simulink library "DCAC_Converter"  (R2018b)
settings: Solver=VariableStepAuto  StartTime=0.0  StopTime=10.0  RelTol=1e-3
settings Model: Creator=Tony  LastModifiedBy=ga69qig
settings SFSimCC: SimUseLocalCustomCode=off
settings RTWCC: RTWUseLocalCustomCode=off

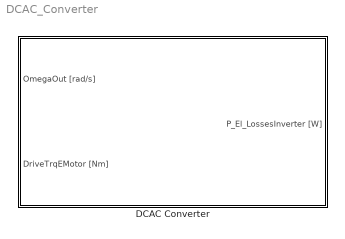
== system DCAC_Converter ==
  DCAC Converter : Subsystem  mask(SB){W_Vektor=[0 10.4719755119660 21.7817090648892 33.0914426178125 44.4011761707357 55.7109097236590 67.0206432765823 78.3303768295055 89.6401103824288 100.949843935352 112.259577488275 123.569311041199 134.879044594122 146.188778147045 157.498511699968 168.808245252892 180.117978805815 191.427712358738 202.737445911661 214.047179464585 225.356913017508 236.666646570431 247.976380123354 259.286113676278 270.595847229201 281.905580782124 293.215314335047 304.525047887971 315.834781440894 327.144514993817 338.454248546740 349.763982099664 361.073715652587 372.383449205510 383.693182758433 395.002916311357 406.312649864280 417.622383417203 428.932116970126 440.241850523050 451.551584075973 462.861317628896 474.171051181819 485.480784734743 496.790518287666 508.100251840589 519.409985393512 530.719718946436 542.029452499359 553.339186052282 564.648919605206 575.958653158129 587.268386711052 598.578120263975 609.887853816898 621.197587369822 632.507320922745 643.817054475668 655.126788028592 666.436521581515 677.746255134438], M_Vektor_motgen=[0 1 2 3 4 5 6 7 8 9 10 11 12 13 14 15 16 17 18 19 20 21 22 23 24 25 26 27 28 29 30 31 32 33 34 35 36 37 38 39 40 41 42 43 44 45 46 47 48 49 50 51 52 53 54 55 56 57 58 59 60 61 62 63 64 65 66 67 68 69 70 71 72 73 74 75 76 77 78 79 80 81 82 83 84 85 86 87 88 89 90 91 92 93 94 95 96 97 98 99 100 101 102 103 104 105 106 107 108 109 110 111 112 113 114 115 116 117 118 119 120 121 122 123 124 125 126 127 128 129 130], P_Loss=[0 0 0 0 0 0 0 0 0 0 0 0 0 0 0 0 0 0 0 0 0 0 0 0 0 0 0 0 0 0 0 0 0 0 0 0 0 0 0 0 0 0 0 0 0 0 0 0 0 0 0 0 0 0 0 0 0 0 0 0 0 0 0 0 0 0 0 0 0 0 0 0 0 0 0 0 0 0 0 0 0 0 0 0 0 0 0 0 0 0 0 0 0 0 0 0 0 0 0 0 0 0 0 0 0 0 0 0 0 0 0 0 0 0 0 0 0 0 0 0 0 0 0 0 0 0 0 0 0 0 0;0 82 70 84 90 100 106 112 101 115 122 130 144 146 153 162 154 169 188 198 202 216 231 236 247 260 271 279 293 309 316 326 335 353 373 392 407 427 437 460 475 478 493 505 523 529 551 565 570 582 598 616 631 647 665 682 700 716 730 726 743 763 780 805 824 840 861 884 903 919 947 960 981 995 1018 1041 1062 1086 1110 1130 1152 1170 1188 1211 1237 1259 1280 1302 1323 1344 1369 1392 1412 1440 1460 1493 1518 1540 1568 1594 1617 1646 1670 1709 1743 1769 1791 1825 1856 1881 1938 2212 3001 3444 3441 3510 3626 3825 3876 3879 3957 4140 4177 3954 4094 3971 3839 3839 3839 3839 3839;0 61 78 75 74 73 81 94 94 97 96 106 120 131 139 145 154 169 180 188 198 206 215 230 242 254 265 268 286 302 306 318 344 370 384 399 410 423 438 458 483 500 512 520 528 539 554 573 589 600 614 632 645 655 678 691 714 720 739 748 763 777 787 809 833 829 860 887 913 937 949 962 976 988 1007 1032 1049 1076 1095 1118 1143 1168 1192 1212 1231 1256 1293 1323 1337 1356 1387 1406 1427 1456 1469 1496 1515 1558 1577 1607 1643 1675 1694 1710 1739 1772 1805 1832 1870 1893 1924 1942 1976 1999 2049 2640 3767 4034 4108 4084 4241 4351 4407 4486 4544 4620 3839 3839 3839 3839 3839;0 70 71 95 83 94 92 96 105 107 112 125 141 143 150 153 165 176 190 203 218 233 240 245 253 260 274 285 304 329 341 352 358 365 379 403 424 444 460 472 483 499 525 535 543 561 575 589 597 611 632 643 656 664 677 700 719 731 742 759 777 794 814 839 858 870 892 917 938 953 968 987 1008 1022 1035 1055 1085 1111 1129 1151 1176 1192 1213 1240 1276 1296 1325 1348 1369 1387 1405 1432 1465 1493 1507 1525 1558 1586 1614 1642 1663 1683 1718 1753 1777 1801 1832 1860 1893 1925 1956 1984 2007 2030 2062 2093 2124 2160 2187 2222 2252 2304 2714 4353 4916 3997 3839 3839 3839 3839 3839;0 74 50 130 190 192 101 114 128 71 125 147 164 97 157 185 186 201 216 227 232 238 241 252 264 279 293 306 320 335 355 350 365 394 396 405 423 436 452 468 481 497 508 518 532 545 554 569 588 604 613 625 645 667 677 690 709 726 745 765 780 791 803 829 843 855 881 897 912 926 942 967 994 1017 1036 1056 1073 1104 1121 1152 1181 1210 1240 1264 1282 1303 1323 1349 1371 1396 1415 1439 1469 1495 1515 1540 1563 1591 1625 1648 1677 1706 1736 1764 1793 1824 1842 1877 1912 1945 1975 2002 2024 2048 2081 2116 2143 2180 2207 2259 2278 2340 2348 2402 2412 3130 3839 3839 3839 3839 3839;0 97 63 80 77 71 70 92 102 101 123 143 135 155 167 123 148 166 185 200 226 242 265 255 265 280 315 323 318 335 346 366 381 399 417 422 439 455 469 485 498 512 525 539 550 574 587 589 608 620 642 662 668 685 705 718 725 738 758 776 792 805 834 852 859 885 897 923 947 967 985 998 1012 1023 1052 1079 1100 1125 1143 1167 1187 1214 1253 1276 1309 1333 1360 1375 1400 1424 1445 1464 1482 1504 1536 1562 1591 1615 1648 1680 1708 1734 1763 1796 1819 1825 1852 1870 1910 1946 1979 2013 2048 2088 2118 2153 2189 2216 2239 2276 2311 2337 2377 2430 2439 3130 3839 3839 3839 3839 3839;0 54 47 58 68 60 51 67 76 84 98 114 113 116 128 138 140 157 175 171 180 195 214 221 231 239 258 265 274 290 315 334 355 377 405 415 432 449 467 482 502 518 521 532 552 558 572 584 600 622 634 651 666 679 694 714 726 740 762 782 800 820 833 853 876 894 914 931 953 971 981 991 1011 1036 1068 1088 1111 1128 1142 1166 1197 1229 1255 1273 1304 1348 1379 1414 1440 1454 1475 1496 1514 1537 1564 1589 1611 1605 1652 1678 1706 1735 1768 1805 1835 1862 1903 1936 1962 2002 2036 2057 2079 2113 2149 2183 2212 2244 2285 2323 2355 2386 2410 2437 2457 3130 3839 3839 3839 3839 3839;0 78 78 96 96 93 93 106 115 120 127 134 146 157 157 161 179 196 182 188 211 212 224 245 260 287 306 309 317 325 338 356 376 399 405 416 447 470 487 494 492 494 517 534 542 561 575 584 604 625 635 656 668 681 703 723 742 765 786 804 816 829 843 864 889 904 916 929 942 962 992 1019 1036 1061 1082 ...(+31348 chars)], LocalSampleTime=-1}
      mask prompts: W_Vektor "Reference Omega Vector [1xN]"; M_Vektor_motgen "Reference Torque Vector [1xM]"; P_Loss "Tabled Electric Power Losses [NxM]"; LocalSampleTime "Local System Sample-Time [s]"
      mask help:
      | <Author> Tony Weiss, Benedikt Danquah based on Wacker [1], [2], [3] </Author>
      | <Date> 16/04/2018</Date>
      |
      | <Description>
      | Calculates the electric power losses of the DCAC Converter via Lookup-Table depending on current motor torque and rotational speed. Default values are from the NEmo 100V E-Motor.
      | </Description>
      mask init:
      | GlobalSampleTime = CalcGlobalSampleTime(LocalSampleTime);
      mask Help:
      | <Parameters>
      | Reference Omega Vector [1xN]
      | Reference Torque Vector [1xM]
      | Tabled Electric Power Losses [NxM]
      | 
      | with M,N = ∈ {ℕ}
      | Local System Sample-Time [s]
      | 	<Min> GlobalSampleTime </Min>
      | Global Sample-Time [s]
      | </Parameters>
      | 
      | <Inputs>
      | OmegaOut [rad/s]
      | DriveTrqEMotor [Nm]
      | </Inputs>
      | 
      | <Outputs>
      | P_El_LossesInverter [W]
      | </Outputs>
      | 
      | <Sources>
      | [1] P. Wacker, L. Wheldon, M. Sperlich, J. Adermann, and M. Lienkamp, “Influence of active battery switching on the drivetrain efficiency of electric vehicles,” in 2017 IEEE Transportation Electrification Conference (ITEC), Chicago, 2017, pp. 33–38.
      | [2] P. Wacker, J. Adermann, B. Danquah, and M. Lienkamp, “Efficiency determination of active battery switching technology on roller dynamometer,” in Twelfth International Conference on Ecological Vehicles and Renewable Energies, Monaco, 2017, pp. 1–7.
      | [3] P. Wacker, “Effizienzsteigerung im Antriebsstrang von Elektrofahrzeugen mittels aktiver Batteriepackverschaltung,” Dissertation, Institute of Automotive Technology, Technical University Munich, Munich, 2018.
      | </Sources>
      mask TypeOptions LocalSampleTime: OmegaOut [rad//s]/SampleTime | DriveTrqEMotor [Nm]/SampleTime
      mask DialogControl DescHelpVar Prompt: Documentation:
      mask DialogControl Control4 Prompt: %<MaskHelp>
      mask DialogControl show_plot Prompt: Plot Power Losses
      mask DialogControl show_plot Callback:
      | current_path_inverter = gcb;
      | InitPlotInverter(current_path_inverter);
      mask DialogControl rest_default Prompt: Restore Default Data
      mask DialogControl rest_default Callback: ParaFile_DCAC_Converter
      mask DialogControl Container4 Prompt: Sample Time
      mask Display:
      | [picturexpos,pictureypos,picturewidth,pictureheight] = ...
      |     CalcBlockPicturePosition(gcb,1,0.1,0.1,100,100); % calculating picture position depending on Block size and minimum margin size
      | image('DCAC_Converter.svg',[picturexpos pictureypos picturewidth pictureheight])% plot picture to block

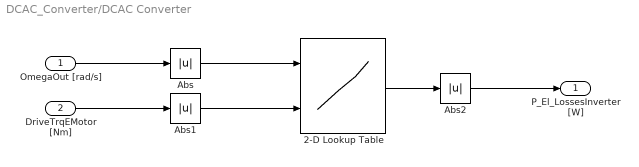
== system DCAC_Converter/DCAC Converter ==
  OmegaOut [rad/s] : Inport  SampleTime=LocalSampleTime
  DriveTrqEMotor [Nm] : Inport  Port=2  SampleTime=LocalSampleTime
  2-D Lookup Table : Lookup_n-D  BreakpointsForDimension1=W_Vektor  BreakpointsForDimension2=M_Vektor_motgen  Table=P_Loss  InternalRulePriority=Speed  RndMeth=Simplest  InputSameDT=on
  Abs : Abs
  Abs1 : Abs
  Abs2 : Abs
  P_El_LossesInverter [W] : Outport  SampleTime=GlobalSampleTime
  wires:
  Abs2/1 -> P_El_LossesInverter [W]/1
  Abs1/1 -> 2-D Lookup Table/2
  Abs/1 -> 2-D Lookup Table/1
  2-D Lookup Table/1 -> Abs2/1
  OmegaOut [rad/s]/1 -> Abs/1
  DriveTrqEMotor [Nm]/1 -> Abs1/1
